simulink model "ruzgar_navigason_sim"  (R2024b)
settings: Solver=VariableStepAuto  StartTime=0.0  StopTime=inf  RelTol=1e-3
settings Model: Creator=ercu  LastModifiedBy=ercu

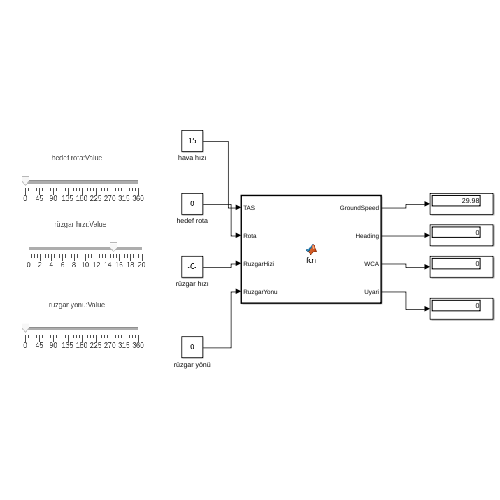
[thumbnail: Simulink's stored preview of the top-level diagram]
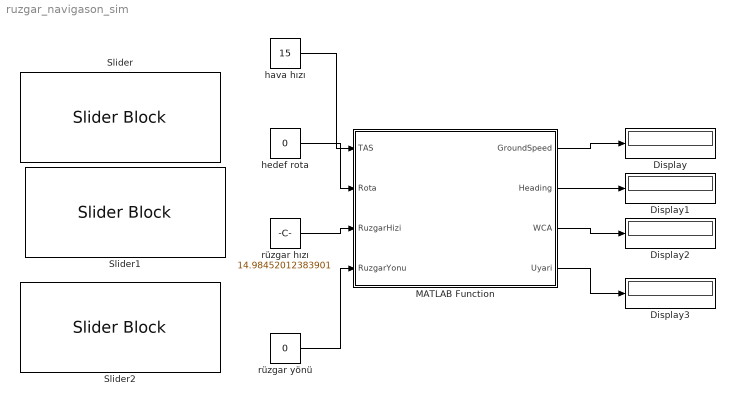
== system ruzgar_navigason_sim ==
  Display{,1..3} (4 alike) : Display
  MATLAB Function : MATLAB Function  TreatAsAtomicUnit=on
  Slider : SliderBlock  ScaleMax=360
  Slider1 : SliderBlock  ScaleMax=20
  Slider2 : SliderBlock  ScaleMax=360
  hava hızı : Constant  Value=15
  hedef rota : Constant  Value=0
  rüzgar hızı : Constant  Value=14.98452012383901
  rüzgar yönü : Constant  Value=0
  wires:
  hava hızı/1 -> MATLAB Function/1(TAS)
  hedef rota/1 -> MATLAB Function/2(Rota)
  rüzgar hızı/1 -> MATLAB Function/3(RuzgarHizi)
  rüzgar yönü/1 -> MATLAB Function/4(RuzgarYonu)
  MATLAB Function/1(GroundSpeed) -> Display/1
  MATLAB Function/2(Heading) -> Display1/1
  MATLAB Function/3(WCA) -> Display2/1
  MATLAB Function/4(Uyari) -> Display3/1

== matlab function ruzgar_navigason_sim/MATLAB Function ==
  data: TAS input; GroundSpeed output; Rota input; RuzgarHizi input; RuzgarYonu input; Heading output; WCA output; Uyari output
function [GroundSpeed, Heading, WCA, Uyari] = fcn(TAS, Rota, RuzgarHizi, RuzgarYonu)
    % Bu fonksiyon Ruzgar Ucgeni hesabini yapar
    
    % 1. Aci Donusumleri (Derece -> Radyan)
    % Ruzgarin "Gittigi" yonu bulmak icin 180 ekliyoruz
    ruzgar_rad = deg2rad(RuzgarYonu + 180);
    rota_rad = deg2rad(Rota);
    
    % 2. Ruzgar Bilesenleri
    Wx = RuzgarHizi * sin(ruzgar_rad);
    Wy = RuzgarHizi * cos(ruzgar_rad);
    
    % 3. WCA (Yengecleme Acisi) Hesabi - Sinus Teoremi
    aci_farki = deg2rad(RuzgarYonu - Rota);
    
    % Guvenlik: Eger ruzgar cok hizliysa asin hata verir (complex number)
    if RuzgarHizi >= TAS
        WCA_rad = 0;
        GroundSpeed = 0;
        Heading = Rota;
        Uyari = 1; % TEHLIKE!
    else
        WCA_rad = asin((RuzgarHizi * sin(aci_farki)) / TAS);
        
        % 4. Heading ve Ground Speed
        Heading = Rota + rad2deg(WCA_rad);
        GroundSpeed = TAS * cos(WCA_rad) + RuzgarHizi * cos(aci_farki);
        Uyari = 0; % GUVEVLI
    end
    
    % Cikis WCA (Derece cinsinden gormek icin)
    WCA = rad2deg(WCA_rad);
end
